simulink model "rezervor"  (R2017b)
settings: Solver=VariableStepAuto  StartTime=0.0  StopTime=10.0  RelTol=1e-3
settings Model: Creator=alinvoicu26  LastModifiedBy=alinvoicu26

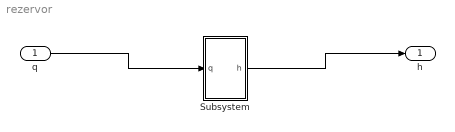
== system rezervor ==
  q : Inport
  Subsystem : Subsystem
  "h " : Outport
  wires:
  q/1 -> Subsystem/1(q)
  Subsystem/1("h ") -> "h "/1

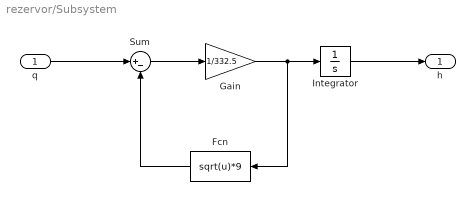
== system rezervor/Subsystem ==
  q : Inport
  Fcn : Fcn  Expr=sqrt(u)*9
  Gain : Gain  Gain=1/332.5
  Integrator : Integrator
  Sum : Sum  Inputs=|+-
  "h " : Outport
  wires:
  q/1 -> Sum/1
  Fcn/1 -> Sum/2
  Integrator/1 -> "h "/1
  Gain/1 -> Fcn/1, Integrator/1
  Sum/1 -> Gain/1
